simulink model "pi_sm_buck_variacao_carga"  (R2016a)
settings: Solver=VariableStepAuto  StartTime=0.0  StopTime=5  RelTol=1e-3
libraries: powerlib x19
settings Model: Creator=jorda  LastModifiedBy=jorda

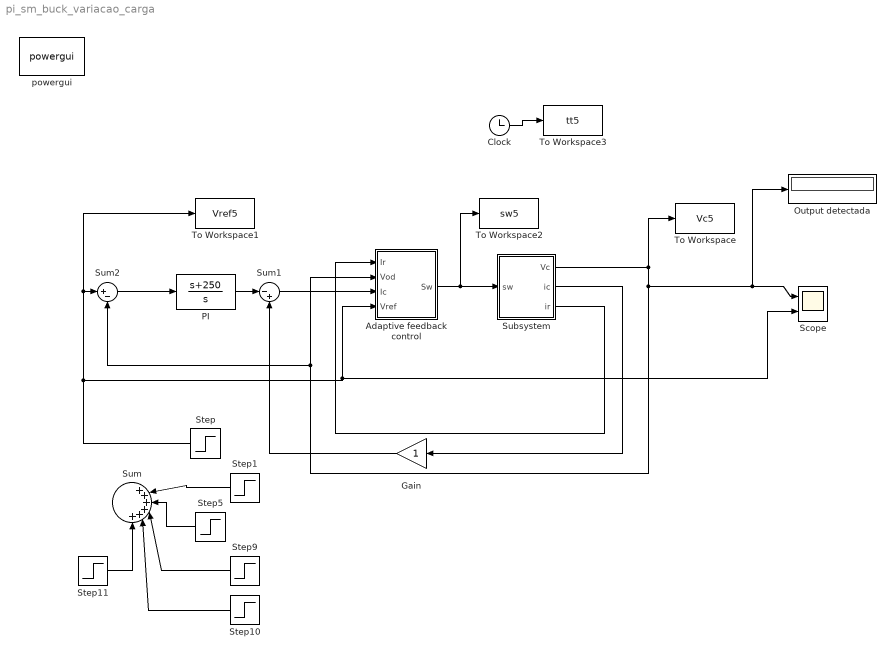
== system pi_sm_buck_variacao_carga ==
  "Adaptive feedback control " : Subsystem
  Clock : Clock
  Gain : Gain
  Output detectada : Display
  PI : TransferFcn  Numerator=[1 250]  Denominator=[1 0]
  Scope : Scope  NumInputPorts=2
  Step : Step  Time=0.5  Before=5  After=5  SampleTime=0
  Step1 : Step  SampleTime=0
  Step10 : Step  Time=2.5  After=-1  SampleTime=0
  Step11 : Step  Time=3  After=2  SampleTime=0
  Step5 : Step  Time=1.5  After=-2  SampleTime=0
  Step9 : Step  Time=2  After=-1  SampleTime=0
  Subsystem : Subsystem
  Sum : Sum  Inputs=|++++++
  Sum1 : Sum  Inputs=|-+
  Sum2 : Sum  Inputs=|+-
  To Workspace : ToWorkspace  VariableName=Vc5  SampleTime=1e-3
  To Workspace1 : ToWorkspace  VariableName=Vref5  SampleTime=1e-3
  To Workspace2 : ToWorkspace  VariableName=sw5  SampleTime=1e-3
  To Workspace3 : ToWorkspace  VariableName=tt5  SampleTime=1e-3
  powergui : powerlib/powergui  Priority=1  SimulationMode=Continuous  SolverType=Tustin/Backward Euler (TBE)  SampleTime=50e-6  frequency=60  SPID=off  DisableSnubberDevices=off  DisableRonSwitches=off  DisableVfSwitches=off  SwTol=0  DisplayEquations=off  Interpol=off  ExternalGateDelay=off  methode=off  Ts=10  FunctionMessages=off  echomessages=off  HookPort=off  EnableUseOfTLC=off  x0status=blocks  frequencyindice=0  Pbase=100e6  ErrMax=1e-4  Iterations=50  UnitsV=kV  UnitsW=MW  buscounter=0  RestoreLinks=warning  ResistiveCurrentMeasurement=off  Frange=[0:2:500]  Ylog=off  Xlog=on  ShowGrid=off  save=off  variable=ZData  structure=0  ZoomFFT=off  StartTime=0.0  cycles=1  DisplayStyle=1  fundamental=60  FreqAxis=off  MaxFrequency=1000  frequencyindicesteady=1  RmsSteady=1  display=off
  wires:
  "Adaptive feedback control "/1(Sw) -> To Workspace2/1, Subsystem/1("sw ")
  Subsystem/2(ic) -> Gain/1
  Subsystem/1(Vc) -> Output detectada/1, Scope/1, Sum2/2, "Adaptive feedback control "/2(Vod), To Workspace/1
  Subsystem/3(ir) -> "Adaptive feedback control "/1(Ir)
  PI/1 -> Sum1/1
  Sum1/1 -> "Adaptive feedback control "/3(Ic)
  Sum2/1 -> PI/1
  Gain/1 -> Sum1/2
  Clock/1 -> To Workspace3/1
  Step1/1 -> Sum/2
  Step5/1 -> Sum/3
  Step9/1 -> Sum/4
  Step10/1 -> Sum/5
  Step11/1 -> Sum/6
  Step/1 -> Scope/2, "Adaptive feedback control "/4(Vref), To Workspace1/1, Sum2/1

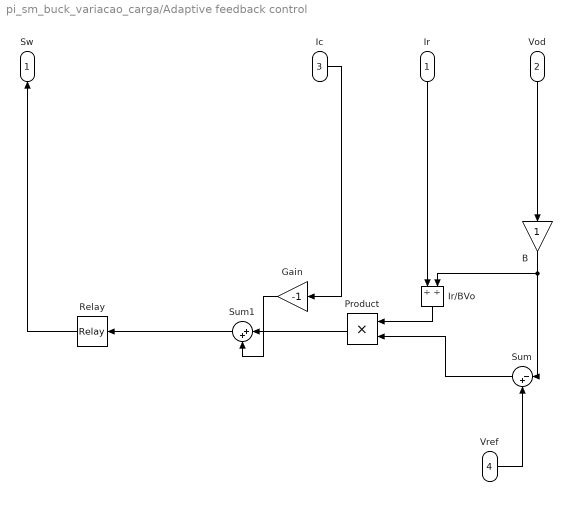
== system pi_sm_buck_variacao_carga/Adaptive feedback control  ==
  Ir : Inport
  Vod : Inport  Port=2
  Ic : Inport  Port=3
  Vref : Inport  Port=4
  B : Gain  ParamDataTypeStr=double  OutDataTypeStr=double
  Gain : Gain  Gain=-1  ParamDataTypeStr=double  OutDataTypeStr=double
  Ir/BVo : Product  Inputs=//
  Product : Product
  Relay : Relay  OnSwitchValue=0.2  OffSwitchValue=-0.2  OutDataTypeStr=double
  Sum : Sum  Inputs=|-+  AccumDataTypeStr=single  OutDataTypeStr=double  InputSameDT=on
  Sum1 : Sum  Inputs=|++  AccumDataTypeStr=double  OutDataTypeStr=double  InputSameDT=on
  Sw : Outport
  wires:
  Product/1 -> Sum1/1
  Ic/1 -> Gain/1
  Gain/1 -> Sum1/2
  Ir/1 -> Ir/BVo/1
  Ir/BVo/1 -> Product/1
  Vod/1 -> B/1
  B/1 -> Ir/BVo/2, Sum/1
  Sum/1 -> Product/2
  Vref/1 -> Sum/2
  Sum1/1 -> Relay/1
  Relay/1 -> Sw/1

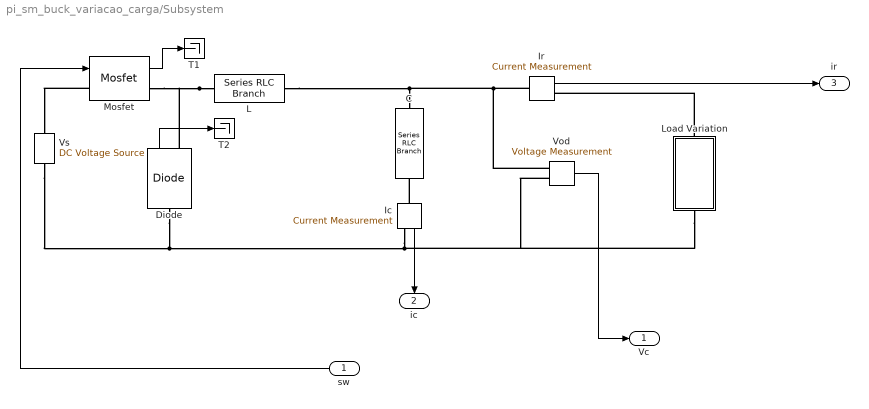
== system pi_sm_buck_variacao_carga/Subsystem ==
  "sw " : Inport
  C : powerlib/Elements/Series RLC Branch  LConnTagsString=__new0  RConnTagsString=__new0  BranchType=C  Resistance=1  Inductance=1e-3  SetiL0=off  InitialCurrent=0  Capacitance=2000e-6  Setx0=off  InitialVoltage=0  Measurements=None
  Diode : powerlib/Power Electronics/Diode  Ron=0.001  Lon=0  Vf=0.8  IC=0  UseSnubber=off  Rs=500  Cs=250e-9  Measurements=on
  Ic : powerlib/Measurements/Current Measurement  PhasorSimulation=off  OutputType=Complex  PSBequivalent=0
  Ir : powerlib/Measurements/Current Measurement  PhasorSimulation=off  OutputType=Complex  PSBequivalent=0
  L : powerlib/Elements/Series RLC Branch  LConnTagsString=__new0  RConnTagsString=__new0  BranchType=L  Resistance=1  Inductance=2e-3  SetiL0=off  InitialCurrent=0  Capacitance=1e-6  Setx0=off  InitialVoltage=0  Measurements=None
  Load Variation : Subsystem
  Mosfet : powerlib/Power Electronics/Mosfet  Ron=0.1  Lon=0  Rd=0.01  Vfd=0  IC=0  Rs=1e5  Cs=inf  Measurements=on
  T1 : Terminator
  T2 : Terminator
  Vod : powerlib/Measurements/Voltage Measurement  PhasorSimulation=off  OutputType=Complex  PSBequivalent=0
  Vs : powerlib/Electrical Sources/DC Voltage Source  Amplitude=15  Measurements=None
  Vc : Outport
  ic : Outport  Port=2
  ir : Outport  Port=3
  wires:
  "sw "/1 -> Mosfet/1
  Mosfet/1 -> T1/1
  Ic/1 -> ic/1
  Diode/1 -> T2/1
  Vod/1 -> Vc/1
  Ir/1 -> ir/1
  connections:
  Diode/LConn1 -- Vs/LConn1 -- Load Variation/RConn1 -- Vod/LConn2 -- Ic/RConn1
  Ic/LConn1 -- C/RConn1
  Ir/LConn1 -- Vod/LConn1 -- L/RConn1 -- C/LConn1
  L/LConn1 -- Mosfet/RConn1 -- Diode/RConn1
  Mosfet/LConn1 -- Vs/RConn1
  Load Variation/LConn1 -- Ir/RConn1

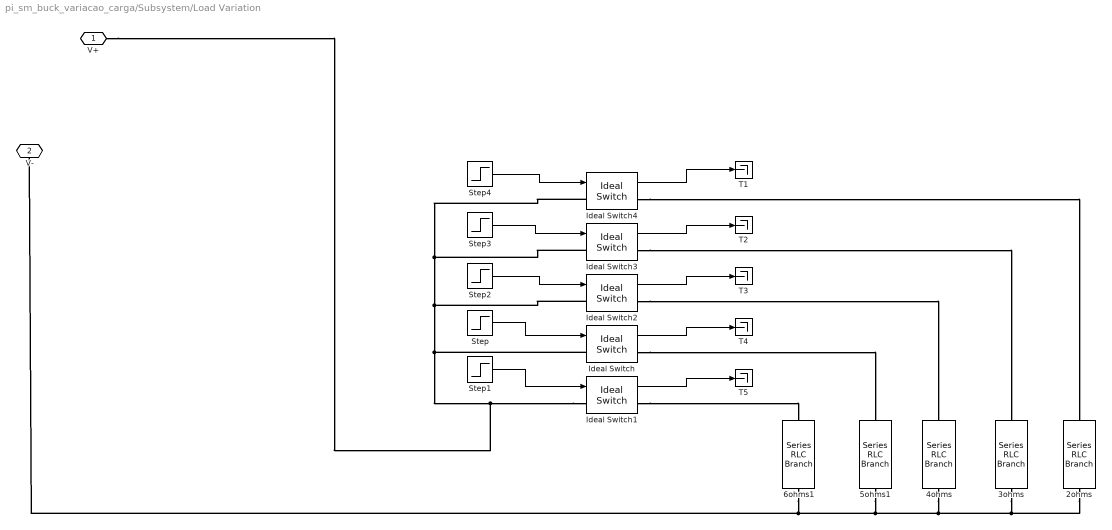
== system pi_sm_buck_variacao_carga/Subsystem/Load Variation ==
  2ohms : powerlib/Elements/Series RLC Branch  LConnTagsString=__new0  RConnTagsString=__new0  BranchType=R  Resistance=2  Inductance=1e-3  SetiL0=off  InitialCurrent=0  Capacitance=1e-6  Setx0=off  InitialVoltage=0  Measurements=None
  3ohms : powerlib/Elements/Series RLC Branch  LConnTagsString=__new0  RConnTagsString=__new0  BranchType=R  Resistance=3  Inductance=1e-3  SetiL0=off  InitialCurrent=0  Capacitance=1e-6  Setx0=off  InitialVoltage=0  Measurements=None
  4ohms : powerlib/Elements/Series RLC Branch  LConnTagsString=__new0  RConnTagsString=__new0  BranchType=R  Resistance=4  Inductance=1e-3  SetiL0=off  InitialCurrent=0  Capacitance=1e-6  Setx0=off  InitialVoltage=0  Measurements=None
  5ohms1 : powerlib/Elements/Series RLC Branch  LConnTagsString=__new0  RConnTagsString=__new0  BranchType=R  Resistance=5  Inductance=1e-3  SetiL0=off  InitialCurrent=0  Capacitance=1e-6  Setx0=off  InitialVoltage=0  Measurements=None
  6ohms1 : powerlib/Elements/Series RLC Branch  LConnTagsString=__new0  RConnTagsString=__new0  BranchType=R  Resistance=6  Inductance=1e-3  SetiL0=off  InitialCurrent=0  Capacitance=1e-6  Setx0=off  InitialVoltage=0  Measurements=None
  Ideal Switch{,1..4} (5 alike) : powerlib/Power Electronics/Ideal Switch  Ron=0.001  Lon=0  IC=0  Rs=1e5  Cs=inf  Measurements=on
  Step : Step  Time=3  After=4  SampleTime=1e-3
  Step1 : Step  Time=4  After=5  SampleTime=1e-3
  Step2 : Step  Time=2  After=3  SampleTime=1e-3
  Step3 : Step  After=2  SampleTime=1e-3
  Step4 : Step  Before=1  After=0  SampleTime=1e-3
  T{1..5} (5 alike) : Terminator
  V+ : PMIOPort  Port=1  Side=Left
  V- : PMIOPort  Port=2  Side=Right
  wires:
  Step2/1 -> Ideal Switch2/1
  Step4/1 -> Ideal Switch4/1
  Step/1 -> Ideal Switch/1
  Step3/1 -> Ideal Switch3/1
  Step1/1 -> Ideal Switch1/1
  Ideal Switch4/1 -> T1/1
  Ideal Switch3/1 -> T2/1
  Ideal Switch2/1 -> T3/1
  Ideal Switch/1 -> T4/1
  Ideal Switch1/1 -> T5/1
  connections:
  Ideal Switch1/LConn1 -- Ideal Switch3/LConn1 -- Ideal Switch4/LConn1 -- Ideal Switch2/LConn1 -- Ideal Switch/LConn1 -- V+/RConn1
  V-/RConn1 -- 6ohms1/RConn1 -- 5ohms1/RConn1 -- 2ohms/RConn1 -- 3ohms/RConn1 -- 4ohms/RConn1
  Ideal Switch3/RConn1 -- 3ohms/LConn1
  Ideal Switch4/RConn1 -- 2ohms/LConn1
  Ideal Switch1/RConn1 -- 6ohms1/LConn1
  Ideal Switch2/RConn1 -- 4ohms/LConn1
  Ideal Switch/RConn1 -- 5ohms1/LConn1
